simulink model "Project1Part2Op2"  (R2024b)
settings: Solver=ode23tb  StartTime=0  StopTime=25  FixedStep=1  RelTol=1e-3
values from neighbouring files (symbols this model uses):
  A = 1    [Project1Part1Graphs.m]
  w_0 = 1    [Project1Part1Graphs.m]
undefined symbols (not defined in the file or in its folder): B1, B2, J1, J2
settings Model: Creator=btagl  LastModifiedBy=btagl

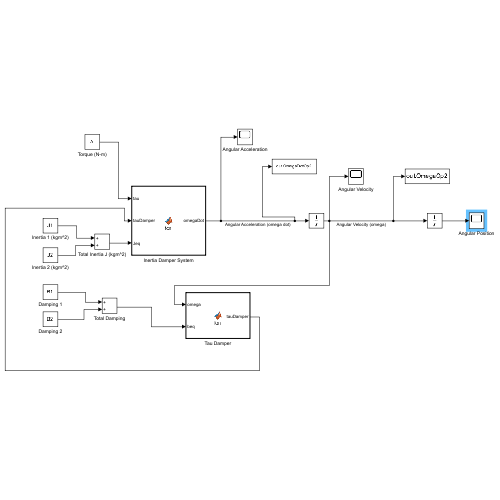
[thumbnail: Simulink's stored preview of the top-level diagram]
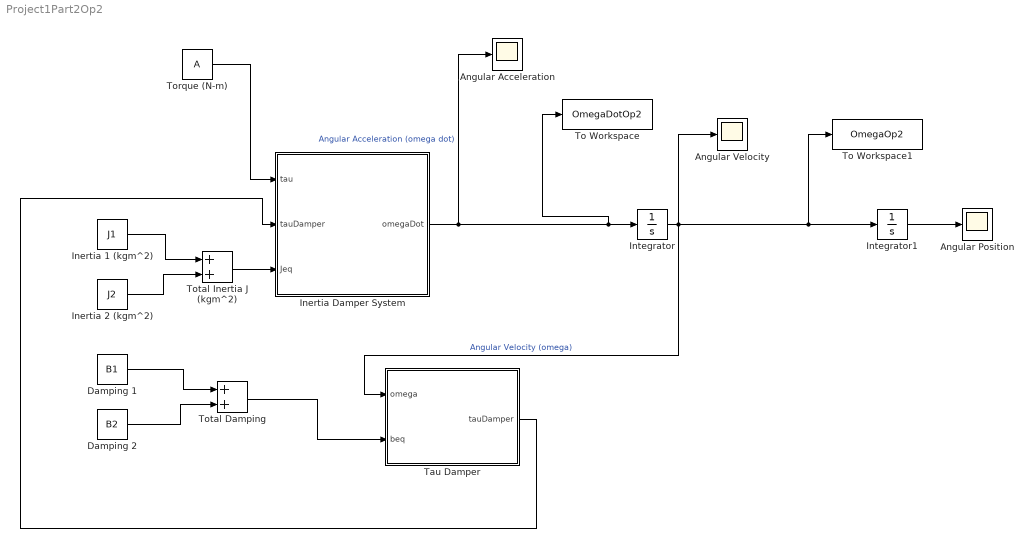
== system Project1Part2Op2 ==
  Angular Acceleration : Scope
  Angular Position : Scope
  Angular Velocity : Scope
  Damping 1 : Constant  Value=B1
  Damping 2 : Constant  Value=B2
  Inertia 1 (kgm^2) : Constant  Value=J1
  Inertia 2 (kgm^2) : Constant  Value=J2
  Inertia Damper System : MATLAB Function  TreatAsAtomicUnit=on
  Integrator : Integrator  InitialCondition=w_0
  Integrator1 : Integrator
  Tau Damper : MATLAB Function  TreatAsAtomicUnit=on
  To Workspace : ToWorkspace  VariableName=OmegaDotOp2  SaveFormat=Timeseries  SampleTime=-1
  To Workspace1 : ToWorkspace  VariableName=OmegaOp2  SaveFormat=Timeseries  SampleTime=-1
  Torque (N-m) : Constant  Value=A
  Total Damping : Sum
  Total Inertia J (kgm^2) : Sum
  wires:
  Inertia 1 (kgm^2)/1 -> Total Inertia J (kgm^2)/1
  Inertia 2 (kgm^2)/1 -> Total Inertia J (kgm^2)/2
  Damping 1/1 -> Total Damping/1
  Damping 2/1 -> Total Damping/2
  Torque (N-m)/1 -> Inertia Damper System/1(tau)
  Total Inertia J (kgm^2)/1 -> Inertia Damper System/3(Jeq)
  Inertia Damper System/1(omegaDot) -> Angular Acceleration/1, To Workspace/1, Integrator/1  "Angular Acceleration (omega dot)"
  Integrator/1 -> Angular Velocity/1, Tau Damper/1(omega), To Workspace1/1, Integrator1/1  "Angular Velocity (omega)"
  Total Damping/1 -> Tau Damper/2(beq)
  Tau Damper/1(tauDamper) -> Inertia Damper System/2(tauDamper)
  Integrator1/1 -> Angular Position/1

== matlab function Project1Part2Op2/Inertia Damper System ==
  data: tau input; tauDamper input; omegaDot output; Jeq input
function omegaDot = fcn(tau, tauDamper, Jeq)

omegaDot = (tau-tauDamper)/Jeq;

== matlab function Project1Part2Op2/Tau Damper ==
  data: omega input; tauDamper output; beq input
function tauDamper = fcn(omega, beq)

tauDamper = omega*beq;
